simulink model "traffic_light_decision"  (R2024b)
settings: Solver=VariableStepAuto  StartTime=0.0  StopTime=10.0  RelTol=1e-3
settings Model: Creator=hadi  LastModifiedBy=hadi

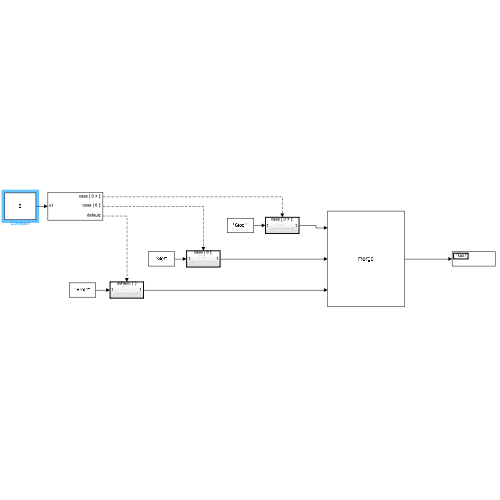
[thumbnail: Simulink's stored preview of the top-level diagram]
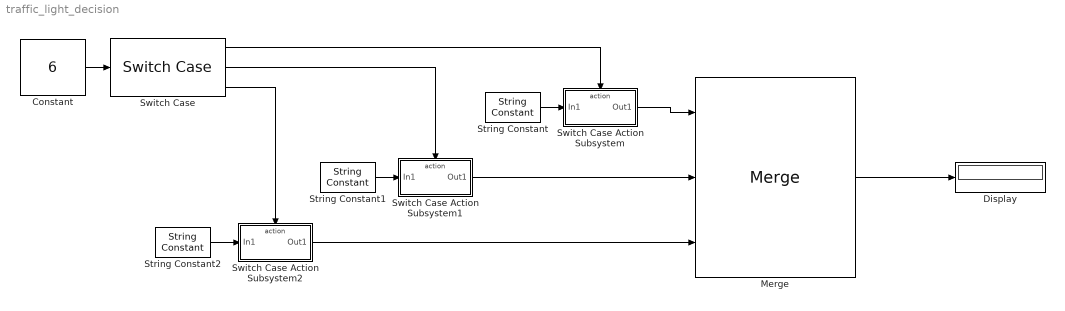
== system traffic_light_decision ==
  Constant : Constant  Value=6
  Display : Display
  Merge : Merge  Inputs=3
  String Constant : StringConstant  String="\"Stop!\""
  String Constant1 : StringConstant  String="\"Go!\""
  String Constant2 : StringConstant  String="\"Error!\""
  Switch Case : SwitchCase  CaseConditions={[3,7],6}
  Switch Case Action Subsystem : Subsystem  TreatAsAtomicUnit=on
  Switch Case Action Subsystem1 : Subsystem  TreatAsAtomicUnit=on
  Switch Case Action Subsystem2 : Subsystem  TreatAsAtomicUnit=on
  wires:
  Constant/1 -> Switch Case/1
  String Constant/1 -> Switch Case Action Subsystem/1(In1)
  String Constant1/1 -> Switch Case Action Subsystem1/1(In1)
  String Constant2/1 -> Switch Case Action Subsystem2/1(In1)
  Switch Case/3 -> Switch Case Action Subsystem2/Action
  Switch Case/2 -> Switch Case Action Subsystem1/Action
  Switch Case/1 -> Switch Case Action Subsystem/Action
  Switch Case Action Subsystem/1(Out1) -> Merge/1
  Switch Case Action Subsystem1/1(Out1) -> Merge/2
  Switch Case Action Subsystem2/1(Out1) -> Merge/3
  Merge/1 -> Display/1

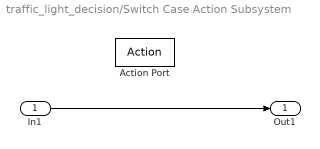
== system traffic_light_decision/Switch Case Action Subsystem ==
  In1 : Inport
  Action Port : ActionPort  ActionPortLabel=case [ 3 7 ]:
  Out1 : Outport
  wires:
  In1/1 -> Out1/1

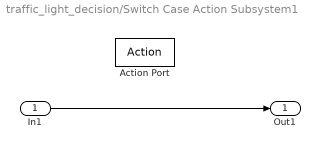
== system traffic_light_decision/Switch Case Action Subsystem1 ==
  In1 : Inport
  Action Port : ActionPort  ActionPortLabel=case [ 6 ]:
  Out1 : Outport
  wires:
  In1/1 -> Out1/1

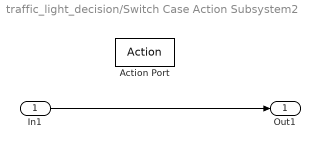
== system traffic_light_decision/Switch Case Action Subsystem2 ==
  In1 : Inport
  Action Port : ActionPort  ActionPortLabel=default:
  Out1 : Outport
  wires:
  In1/1 -> Out1/1
